simulink model "a2_step"  (R2018a)
settings: Solver=VariableStepAuto  StartTime=0.0  StopTime=10.0  RelTol=1e-3
settings Model: Creator=oleksandra  LastModifiedBy=oleksandra

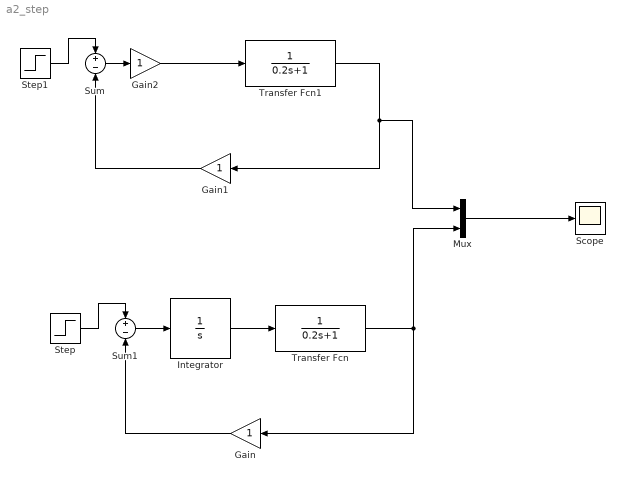
== system a2_step ==
  Gain : Gain
  Gain1 : Gain
  Gain2 : Gain
  Integrator : Integrator
  Mux : Mux  Inputs=2
  Scope : Scope
  Step : Step  SampleTime=0
  Step1 : Step  SampleTime=0
  Sum : Sum  Inputs=+-
  Sum1 : Sum  Inputs=+-
  Transfer Fcn : TransferFcn  Denominator=[0.2 1]
  Transfer Fcn1 : TransferFcn  Denominator=[0.2 1]
  wires:
  Sum/1 -> Gain2/1
  Mux/1 -> Scope/1
  Sum1/1 -> Integrator/1
  Transfer Fcn/1 -> Mux/2, Gain/1
  Integrator/1 -> Transfer Fcn/1
  Step1/1 -> Sum/1
  Gain1/1 -> Sum/2
  Step/1 -> Sum1/1
  Gain/1 -> Sum1/2
  Transfer Fcn1/1 -> Mux/1, Gain1/1
  Gain2/1 -> Transfer Fcn1/1
